simulink model "x3_myfoc_transform"  (R2025b)
settings: Solver=ode23t  StartTime=0.0  StopTime=2  FixedStep=my_Ts  RelTol=1e-3
values from neighbouring files (symbols this model uses):
  Jx = 0.0000005    (= 5e-07)    [foc_para.m]
  Tpwm = 4000-1    (= 3999)    [foc_para.m]
  Ts = 1/SwitchFrequency    (= 5e-05)    [foc_para.m]
  vbus = 12    [foc_para.m]
undefined symbols (not defined in the file or in its folder): DiscIntNeverNeededParam, my_Ts
libraries: ee_lib x11, fl_lib x9, nesl_utility x9, simulink x1
settings Model: Creator=disnox  LastModifiedBy=yolo
settings DataIOCC: ReturnWorkspaceOutputs=off
settings DebuggingCC: SaveWithParameterizedLinksMsg=none  ParameterPrecisionLossMsg=none
settings HardwareCC: ProdBitPerPointer=32.0  ProdBitPerSizeT=32.0  ProdBitPerPtrDiffT=32.0  ProdLargestAtomicInteger=Long  ProdLargestAtomicFloat=Double  ProdWordSize=32.0  ProdHWDeviceType=ARM Compatible->ARM Cortex-M
settings RTWCC: GPUComputeCapability=3.5

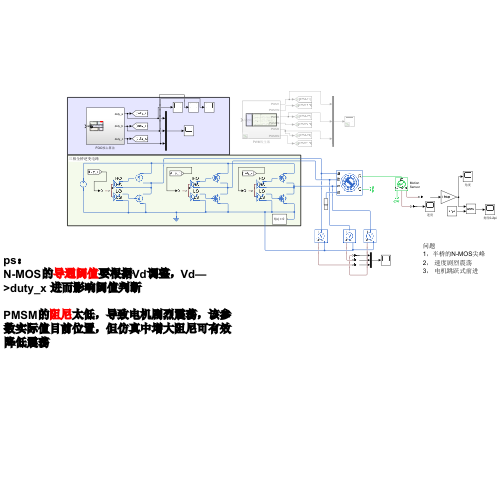
[thumbnail: Simulink's stored preview of the top-level diagram]
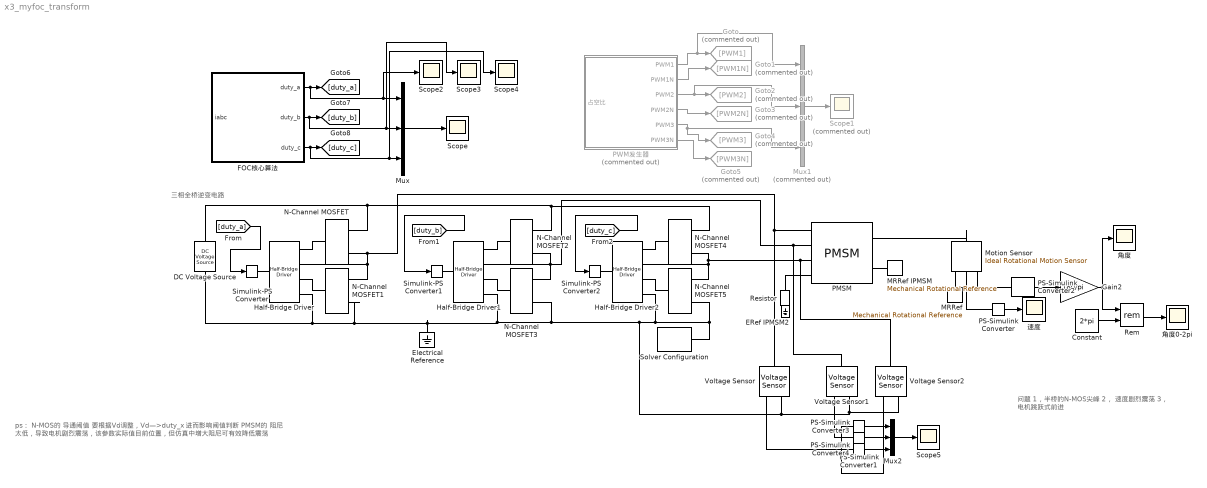
== system x3_myfoc_transform ==
  note: 问题
      | 1，半桥的N-MOS尖峰
      | 2， 速度剧烈震荡
      | 3， 电机跳跃式前进
  note: ps：
      | N-MOS的 导通阈值 要根据Vd调整，Vd—>duty_x 进而影响阈值判断
      |
      | PMSM的 阻尼 太低，导致电机剧烈震荡，该参数实际值目前位置，但仿真中增大阻尼可有效降低震荡
  note: 三相全桥逆变电路
  Constant : Constant  Value=2*pi
  DC Voltage Source : ee_lib/Additional Components/SPICE Sources/DC Voltage Source  DC=12 V
  ERef IPMSM2 : fl_lib/Electrical/Electrical Elements/Electrical Reference
  Electrical Reference : fl_lib/Electrical/Electrical Elements/Electrical Reference
  FOC核心算法 : Subsystem
  Gain2 : Gain  Gain=180/pi
  Goto : Goto  Commented=on  GotoTag=PWM1
  Goto1 : Goto  Commented=on  GotoTag=PWM1N
  Goto2 : Goto  Commented=on  GotoTag=PWM2
  Goto3 : Goto  Commented=on  GotoTag=PWM2N
  Goto4 : Goto  Commented=on  GotoTag=PWM3
  Goto5 : Goto  Commented=on  GotoTag=PWM3N
  Half-Bridge Driver : ee_lib/Semiconductors & Converters/Half-Bridge Driver  port_option=ee.enum.controlport.ps  uHigh=2.0 V  uLow=0.8 V  uHighValue=0.6  uLowValue=0.4  vHigh=12 V  vLow=0 V  tpLH=50 ns  tdLH=5 us  tpHL=50 ns  tdHL=5 us  parameterization=ee.enum.semiconductors.gateDriverParam.outputImpedance  rHigh=50 Ohm  rLow=50 Ohm  tRise=20 ns  tFall=20 ns  cLoad=10 nF  ZonTime_specify=off  ZonTime_priority=None  ZonTime=0 s  ZoffTime_specify=off  ZoffTime_priority=None  ZoffTime=0 s  power_dissipated_high_side_specify=off  power_dissipated_high_side_priority=None  power_dissipated_high_side=0 W  power_dissipated_high_side_nominal_specify=off  power_dissipated_high_side_nominal_value=1  power_dissipated_high_side_nominal_unit=W  power_dissipated_low_side_specify=off  power_dissipated_low_side_priority=None  power_dissipated_low_side=0 W  power_dissipated_low_side_nominal_specify=off  power_dissipated_low_side_nominal_value=1  power_dissipated_low_side_nominal_unit=W
      settings: InternalSimscapePortConfiguration="{\"Bottom\":[],\"Left\":[{\"id\":\"u\",\"label\":\"u\",\"type\":\"input\"}],\"Right\":[{\"id\":\"HO\",\"label\":\"HO\",\"type\":\"foundation.electrical.electrical\"},{\"id\":\"HS\",\"label\":\"HS\",\"type\":\"foundation.electrical.electrical\"},{\"id\":\"LO\",\"label\":\"LO\",\"type\":\"foundation.electrical.electrical\"},{\"id\":\"LS\",\"label\":\"LS\",\"type\":\"foundation.electrical.electrical\"}],\"Top\":[]}"
  Half-Bridge Driver1 : ee_lib/Semiconductors & Converters/Half-Bridge Driver  port_option=ee.enum.controlport.ps  uHigh=2.0 V  uLow=0.8 V  uHighValue=0.6  uLowValue=0.4  vHigh=12 V  vLow=0 V  tpLH=50 ns  tdLH=5 us  tpHL=50 ns  tdHL=5 us  parameterization=ee.enum.semiconductors.gateDriverParam.outputImpedance  rHigh=50 Ohm  rLow=50 Ohm  tRise=20 ns  tFall=20 ns  cLoad=10 nF  ZonTime_specify=off  ZonTime_priority=None  ZonTime=0 s  ZoffTime_specify=off  ZoffTime_priority=None  ZoffTime=0 s  power_dissipated_high_side_specify=off  power_dissipated_high_side_priority=None  power_dissipated_high_side=0 W  power_dissipated_high_side_nominal_specify=off  power_dissipated_high_side_nominal_value=1  power_dissipated_high_side_nominal_unit=W  power_dissipated_low_side_specify=off  power_dissipated_low_side_priority=None  power_dissipated_low_side=0 W  power_dissipated_low_side_nominal_specify=off  power_dissipated_low_side_nominal_value=1  power_dissipated_low_side_nominal_unit=W
      settings: InternalSimscapePortConfiguration="{\"Bottom\":[],\"Left\":[{\"id\":\"u\",\"label\":\"u\",\"type\":\"input\"}],\"Right\":[{\"id\":\"HO\",\"label\":\"HO\",\"type\":\"foundation.electrical.electrical\"},{\"id\":\"HS\",\"label\":\"HS\",\"type\":\"foundation.electrical.electrical\"},{\"id\":\"LO\",\"label\":\"LO\",\"type\":\"foundation.electrical.electrical\"},{\"id\":\"LS\",\"label\":\"LS\",\"type\":\"foundation.electrical.electrical\"}],\"Top\":[]}"
  Half-Bridge Driver2 : ee_lib/Semiconductors & Converters/Half-Bridge Driver  port_option=ee.enum.controlport.ps  uHigh=2.0 V  uLow=0.8 V  uHighValue=0.6  uLowValue=0.4  vHigh=12 V  vLow=0 V  tpLH=50 ns  tdLH=5 us  tpHL=50 ns  tdHL=5 us  parameterization=ee.enum.semiconductors.gateDriverParam.outputImpedance  rHigh=50 Ohm  rLow=50 Ohm  tRise=20 ns  tFall=20 ns  cLoad=10 nF  ZonTime_specify=off  ZonTime_priority=None  ZonTime=0 s  ZoffTime_specify=off  ZoffTime_priority=None  ZoffTime=0 s  power_dissipated_high_side_specify=off  power_dissipated_high_side_priority=None  power_dissipated_high_side=0 W  power_dissipated_high_side_nominal_specify=off  power_dissipated_high_side_nominal_value=1  power_dissipated_high_side_nominal_unit=W  power_dissipated_low_side_specify=off  power_dissipated_low_side_priority=None  power_dissipated_low_side=0 W  power_dissipated_low_side_nominal_specify=off  power_dissipated_low_side_nominal_value=1  power_dissipated_low_side_nominal_unit=W
      settings: InternalSimscapePortConfiguration="{\"Bottom\":[],\"Left\":[{\"id\":\"u\",\"label\":\"u\",\"type\":\"input\"}],\"Right\":[{\"id\":\"HO\",\"label\":\"HO\",\"type\":\"foundation.electrical.electrical\"},{\"id\":\"HS\",\"label\":\"HS\",\"type\":\"foundation.electrical.electrical\"},{\"id\":\"LO\",\"label\":\"LO\",\"type\":\"foundation.electrical.electrical\"},{\"id\":\"LS\",\"label\":\"LS\",\"type\":\"foundation.electrical.electrical\"}],\"Top\":[]}"
  MRRef : fl_lib/Mechanical/Rotational Elements/Mechanical Rotational Reference
  MRRef IPMSM : fl_lib/Mechanical/Rotational Elements/Mechanical Rotational Reference
  Motion Sensor : fl_lib/Mechanical/Mechanical Sensors/Ideal Rotational Motion Sensor  reference=foundation.enum.MeasurementReference.difference  acceleration_port=false  velocity_port=true  position_port=true  wrap_angle=false  offset=0 deg
  Mux : Mux  Inputs=3
  Mux1 : Mux  Commented=on  Inputs=3
  Mux2 : Mux  Inputs=3
  N-Channel MOSFET{,1..5} (6 alike) : ee_lib/Semiconductors & Converters/N-Channel MOSFET  paramTerminal=ee.enum.mosfet.numberOfTerminals.three  parameterization=ee.enum.mosfet.parameterization.datasheet  Beta=5.0 A/V^2  Rds=0.025 Ohm  Id=6.0 A  Vgs=10 V  Vth=1.7 V  Vth0=1.7 V  lam=0 1/V  gamma_vth=0.5 V^(1/2)  phib=0.5 V  Vth1=1.9071 V  Vbs1=-1 V  Vth2=2.066 V  Vbs2=-2 V  Tmeas=25 degC  Vgs_vec=[-1, -.5, 2, 3, 4, 5] V  Vds_vec=[0, 2, 4, 8, 12, 16, 20] V  Vbs_vec=[0, -4, -6, -12] V  T_vec=[25, 125] degC  Vth_vec=[.4, 1.2, 1.4, 1.45] V  Vth_mat=[.4, .35; 1.2, 1.15; 1.4, 1.35; 1.45, 1.4] V  Ids_mat=[0, 0, 0, 0, 0, 0, 0; 0, 0, 0, 0, 0, 0, 0; 0, .003, .0038, .0043, .0046, .0048, .0049; 0, .0055, .008, .009, .0095, .01, .0101; 0, .0115, .016, .018, .019, .0195, .02; 0, .0152, .0225, .0265, .028, .0295, .03] A  Ids_mat0=[0, 0, 0, 0, 0, 0, 0; 0, 0, 0, 0, 0, 0, 0; 0, .003, .0038, .0043, .0046, .0048, .0049; 0, .0055, .008, .009, .0095, .01, .0101; 0, .0115, .016, .018, .019, .0195, .02; 0, .0152, .0225, .0265, .028, .0295, .03] A  Ids_mat_3D=zeros(6, 7, 2) A  Ids_mat_3D0=zeros(6, 7, 2) A  IV_table_symmetry=ee.enum.mosfet.symmetricNIV.no  RS=0.0001 Ohm  RD=0.01 Ohm  RB=0.001 Ohm  LeadRs=0 Ohm  LeadRd=0 Ohm  LeadRg=0 Ohm  LeadRb=0 Ohm  LS=0 nH  LD=0 nH  LG=0 nH  LB=0 nH  C_param=ee.enum.mosfet.capacitanceParam.fixedciss  C_GS=270 pF  C_GD=80 pF  C_GB=0 pF  C_DS=0 pF  C_iss=350 pF  C_rss=80 pF  C_oss=0 pF  C_iss_vec=[720, 700, 590, 470, 390, 310] pF  C_rss_vec=[450, 400, 300, 190, 95, 55] pF  C_oss_vec=[900, 810, 690, 420, 270, 170] pF  C_GS_vec=[270, 300, 290, 280, 295, 255] pF  C_GD_vec=[450, 400, 300, 190, 95, 55] pF  C_GB_vec=[270, 300, 290, 280, 295, 255] pF  C_Vgs_vec=0 V  C_DS_vec=[450, 410, 390, 230, 175, 115] pF  C_Vds_vec=[.1, .3, 1, 3, 10, 30] V  V_GS_for_cap_data=0 V  charge_linearity_param=ee.enum.mosfet.cgdLinearity.constant  C_OX=200 pF  V_C_OX=-0.5 V  charge_linearity_param_vgb=ee.enum.mosfet.cgbLinearity.instantly  charge_linearity_param_with_vgb=ee.enum.mosfet.cgbLinearityWithSeparateCgb.instantly  Di_param=ee.enum.mosfet.diodeParam.no  IsDiode=1e-12 A  Vbi=0.6 V  n=1  Cj0Diode=0 pF  TT=50e-9 s  Tmeas_dio=25 degC  TableTypeNoT=ee.enum.mosfet.tableType.IfMat  TableType=ee.enum.diode.tableType.IfMat  IfVec=[.07, .12, .19, 1.75, 4.24, 7.32, 11.2] A  IfMat=[.07, .12, .19, 1.75, 4.24, 7.32, 11.2; .16, .3, .72, 2.14, 4.02, 6.35, 9.12] A  VfVecV=[.9, 1.15, 1.25, 1.5, 1.75, 2.17, 2.6, 2.85] V  VfMatV=[.9, 1.15, 1.25, 1.5, 1.75, 2.17, 2.6, 2.85; .58, .68, .75, 1.1, 1.38, 1.77, 2.27, 2.7] V  TjVec=[25, 125] degC  VfVec=[.5, .7, .9, 1.3, 1.7, 2.1, 2.5] V  IfVecV=[.1, .2, .5, 1, 2, 4, 7, 10] A  diode_Goff=1e-12 1/Ohm  prmDatasheet=ee.enum.temperatureParameterization.none  prmEquCoeff=ee.enum.temperatureParameterization.none  dVth_dT=-6 mV/K  dVth0_dT=-6 mV/K  Rds_T2=0.037 Ohm  BEXDatasheet=-1.5  BEXEquCoeff=-1.5  etaisDatasheet=3  etaisEquCoeff=3  Tmeas2=125 degC  etaisTabulated=3  TdeviceDatasheet=25 degC  TdeviceEquCoeff=25 degC  TdeviceTabulated=25 degC  i_g_specify=off  i_g_priority=None  i_g=0 A  i_g_nominal_specify=off  i_g_nominal_value=1  i_g_nominal_unit=A  i_d_specify=off  i_d_priority=None  i_d=0 A  i_d_nominal_specify=off  i_d_nominal_value=1  i_d_nominal_unit=A  i_b_specify=off  i_b_priority=None  i_b=0 A  i_b_nominal_specify=off  i_b_nominal_value=1  i_b_nominal_unit=A  voltage_gs_specify=off  voltage_gs_priority=None  voltage_gs=0 V  voltage_gs_nominal_specify=off  voltage_gs_nominal_value=1  voltage_gs_nominal_unit=V  voltage_ds_specify=off  voltage_ds_priority=None  voltage_ds=0 V  voltage_ds_nominal_specify=off  voltage_ds_nominal_value=1  voltage_ds_nominal_unit=V  voltage_bs_specify=off  voltage_bs_priority=None  voltage_bs=0 V  voltage_bs_nominal_specify=off  voltage_bs_nominal_value=1  voltage_bs_nominal_unit=V  v_Cgs_specify=off  v_Cgs_priority=High  v_Cgs=0 V  v_Cgs_nominal_specify=off  v_Cgs_nominal_value=1  v_Cgs_nominal_unit=V  v_Cds_specify=off  v_Cds_priority=High  v_Cds=0 V  v_Cds_nominal_specify=off  v_Cds_nominal_value=1  v_Cds_nominal_unit=V  v_Cbs_specify=off  v_Cbs_priority=High  v_Cbs=0 V  v_Cbs_nominal_specify=off  v_Cbs_nominal_value=1  v_Cbs_nominal_unit=V  thermal_network_parameterization=ee.enum.thermalNetworkTopology.junctionCase  Rth=[0, 10] K/W  Rth_Cauer=[1, 3, 10] K/W  Rth_Foster=[.08, .14, .22, .16] K/W  thermal_mass_parameterization=ee.enum.thermalNetwork.timeconstant  thermal_mass=[0, 1] J/K  thermal_mass_Cauer=[.1, .3, 1] J/K  thermal_mass_Foster=[.001, .005, .05, .5] J/K  thermal_time_constant=[0, 10] s  thermal_time_constant_Cauer=[1, 3, 10] s  thermal_time_constant_Foster=[7e-05, .0007, .01, .08] s  thermal_mass_initial_temperatures=[25, 25] degC  thermal_mass_initial_temperatures_Cauer=[25, 25, 25] degC  Tvec_initial_Foster=[25, 25, 25, 25] degC  betaref=18 A/V^2  Vfbref=-1.1 V  gamma=3.5 V^(1/2)  phib2ref=1 V  thesatref=0.4 1/V  alpha=0  Vp=5e-2 V  thesrref=0 1/V  m=8  Tref=25 degC  Rsref=2e-3 Ohm  Rdref=0.17 Ohm  Rgref=8.4 Ohm  Rbref=2e-3 Ohm  Cox=1500 pF  Cgso=100 pF  Cgdo=14 pF  Isref=5.2e-13 A  Cj0=480 pF  Tprm=1  etabet=1.3  Stvfb=5e-4 V/K  Stphib=-8.5e-4 V/K  etasat=1.04  etasr=0.65  etar=0.95  etais=3  Tsim=25 degC  Ig_specify=off  Ig_priority=None  Ig=0 A  Ig_nominal_specify=off  Ig_nominal_value=1  Ig_nominal_unit=nA  Ids_specify=off  Ids_priority=None  Ids=0 A  Ids_nominal_specify=off  Ids_nominal_value=1  Ids_nominal_unit=A  Ib_specify=off  Ib_priority=None  Ib=0 A  Ib_nominal_specify=off  Ib_nominal_value=1  Ib_nominal_unit=uA  V_gs_specify=off  V_gs_priority=None  V_gs=0 V  V_gs_nominal_specify=off  V_gs_nominal_value=1  V_gs_nominal_unit=V  V_ds_specify=off  V_ds_priority=None  V_ds=0 V  V_ds_nominal_specify=off  V_ds_nominal_value=1  V_ds_nominal_unit=V  V_bs_specify=off  V_bs_priority=None  V_bs=0 V  V_bs_nominal_specify=off  V_bs_nominal_value=1  V_bs_nominal_unit=V  QGoverCox_specify=off  QGoverCox_priority=None  QGoverCox=0 V  QGoverCox_nominal_specify=off  QGoverCox_nominal_value=1  QGoverCox_nominal_unit=V  QDoverCox_specify=off  QDoverCox_priority=None  QDoverCox=0 V  QDoverCox_nominal_specify=off  QDoverCox_nominal_value=1  QDoverCox_nominal_unit=V  QBoverCox_specify=off  QBoverCox_priority=None  QBoverCox=0 V  QBoverCox_nominal_specify=off  QBoverCox_nominal_value=1  QBoverCox_nominal_unit=V  T0=[25, 25] degC  T0_Cauer=[25, 25, 25] degC
  PMSM : ee_lib/Electromechanical/Permanent Magnet/PMSM  port_option=ee.enum.threePhasePort.expanded  winding_type=ee.enum.electromech.statorconfiguration.wye  machine_param=ee.enum.pmsm.parameterization.constant  nPolePairs=Np  pmflux_param=ee.enum.pmflux.fluxlinkage  pm_flux_linkage=Flux Wb  torque_constant=0.18 N*m/A  back_emf_constant=0.18 V*s/rad  stator_param=ee.enum.statorparam.LdLqL0  Ld=Ld H  Lq=Lq H  idVec=[-200, 0, 200] A  iqVec=[-200, 0, 200] A  LdMatrix=0.0002 * ones(3, 3) H  LqMatrix=0.0002 * ones(3, 3) H  PmMatrix=0.1 * ones(3, 3) Wb  ktMatrix=0.18 * ones(3, 3) N*m/A  keMatrix=0.18 * ones(3, 3) V*s/rad  L0=0.00016 H  Ls=0.0002 H  Lm=-0.00002 H  Ms=0.00002 H  Rs=Rs Ohm  zero_sequence=ee.enum.park.zerosequence.include  axes_param=ee.enum.rotorangle.daxis  loss_param=ee.enum.ironloss.none  losses_oc=[0, 0, 0] W  losses_sc=[0, 0, 0] W  f_losses=60 Hz  Isc_losses=95 A  J=Jx kg*m^2  lam=0.001 N*m*s/rad  i_d_specify=off  i_d_priority=None  i_d=0 A  i_d_nominal_specify=off  i_d_nominal_value=1  i_d_nominal_unit=A  i_q_specify=off  i_q_priority=None  i_q=0 A  i_q_nominal_specify=off  i_q_nominal_value=1  i_q_nominal_unit=A  torque_specify=off  torque_priority=None  torque=0 N*m  torque_nominal_specify=off  torque_nominal_value=1  torque_nominal_unit=N*m  angular_velocity_specify=off  angular_velocity_priority=High  angular_velocity=0 rpm  angular_velocity_nominal_specify=off  angular_velocity_nominal_value=1  angular_velocity_nominal_unit=rpm  angular_position_specify=off  angular_position_priority=High  angular_position=0 deg  angular_position_nominal_specify=off  angular_position_nominal_value=1  angular_position_nominal_unit=deg  alpha=3.93e-3 1/K  alpha_flux=-0.001 1/K  Tmeas=298.15 K  stator_thermal_mass=100 J/K  rotor_thermal_mass=200 J/K  Rm_percent_rotor=90  Rd_percent_rotor=30  temperatureA_specify=off  temperatureA_priority=High  temperatureA=25 degC  temperatureA_nominal_specify=off  temperatureA_nominal_value=1  temperatureA_nominal_unit=degC  temperatureB_specify=off  temperatureB_priority=High  temperatureB=25 degC  temperatureB_nominal_specify=off  temperatureB_nominal_value=1  temperatureB_nominal_unit=degC  temperatureC_specify=off  temperatureC_priority=High  temperatureC=25 degC  temperatureC_nominal_specify=off  temperatureC_nominal_value=1  temperatureC_nominal_unit=degC  temperatureR_specify=off  temperatureR_priority=High  temperatureR=25 degC  temperatureR_nominal_specify=off  temperatureR_nominal_value=1  temperatureR_nominal_unit=degC
      settings: InternalSimscapePortConfiguration="{\"Bottom\":[],\"Left\":[{\"id\":\"a\",\"label\":\"a\",\"type\":\"foundation.electrical.electrical\"},{\"id\":\"b\",\"label\":\"b\",\"type\":\"foundation.electrical.electrical\"},{\"id\":\"c\",\"label\":\"c\",\"type\":\"foundation.electrical.electrical\"},{\"id\":\"n\",\"label\":\"n\",\"type\":\"foundation.electrical.electrical\"}],\"Right\":[{\"id\":\"R\",\"label\":\"R\",\"type\":\"foundation.mechanical.rotational.rotational\"},{\"id\":\"C\",\"label\":\"C\",\"type\":\"foundation.mechanical.rotational.rotational\"}],\"Top\":[]}"
  PS-Simulink Converter : nesl_utility/PS-Simulink Converter  PhysicalDomain=network_engine_domain  SubClassName=ps_output  LeftPortType=input  RightPortType=output  PseudoPeriodic=off  Frequencies=[]  VectorFormat=inherit  Unit=rad/s  AffineConversion=off
  PS-Simulink Converter1 : nesl_utility/PS-Simulink Converter  PhysicalDomain=network_engine_domain  SubClassName=ps_output  LeftPortType=input  RightPortType=output  PseudoPeriodic=off  Frequencies=[]  VectorFormat=inherit  Unit=inherit  AffineConversion=off
  PS-Simulink Converter2 : nesl_utility/PS-Simulink Converter  PhysicalDomain=network_engine_domain  SubClassName=ps_output  LeftPortType=input  RightPortType=output  PseudoPeriodic=off  Frequencies=[]  VectorFormat=1-D array  Unit=rad  AffineConversion=off
  PS-Simulink Converter3 : nesl_utility/PS-Simulink Converter  PhysicalDomain=network_engine_domain  SubClassName=ps_output  LeftPortType=input  RightPortType=output  PseudoPeriodic=off  Frequencies=[]  VectorFormat=inherit  Unit=inherit  AffineConversion=off
  PS-Simulink Converter4 : nesl_utility/PS-Simulink Converter  PhysicalDomain=network_engine_domain  SubClassName=ps_output  LeftPortType=input  RightPortType=output  PseudoPeriodic=off  Frequencies=[]  VectorFormat=inherit  Unit=inherit  AffineConversion=off
  PWM发生器 : Subsystem  Commented=on
  Rem : Math  Operator=rem
  Resistor : fl_lib/Electrical/Electrical Elements/Resistor  R=1e9 Ohm  i_specify=off  i_priority=None  i=0 A  i_nominal_specify=off  i_nominal_value=1  i_nominal_unit=A  v_specify=off  v_priority=None  v=0 V  v_nominal_specify=off  v_nominal_value=1  v_nominal_unit=V
  Scope{,2..5} (5 alike) : Scope
      Scope settings: ActiveDisplayYMinimum=0.31957804087824193  ActiveDisplayYMaximum=0.68042195912175807  DataLoggingVariableName=ScopeData15
      Scope2 settings: ActiveDisplayYMinimum=-0.37624405782146064  ActiveDisplayYMaximum=1.3678304816261502  DataLoggingVariableName=ScopeData17
      Scope3 settings: ActiveDisplayYMinimum=-0.24057027373037865  ActiveDisplayYMaximum=1.4204530971721079  DataLoggingVariableName=ScopeData18
      Scope4 settings: ActiveDisplayYMinimum=-0.24057027373037865  ActiveDisplayYMaximum=1.4204530971721079  DataLoggingVariableName=ScopeData19
      Scope5 settings: ActiveDisplayYMinimum=-9.0067395854845973  ActiveDisplayYMaximum=21.007224453015507  DataLoggingVariableName=ScopeData21
  Scope1 : Scope  Commented=on
      settings: DataLoggingVariableName=ScopeData14
  Simulink-PS Converter : nesl_utility/Simulink-PS Converter  PhysicalDomain=network_engine_domain  SubClassName=ps_input  LeftPortType=input  RightPortType=output  PseudoPeriodic=off  Frequencies=[]  NoiseDistribution=none  NoiseParameters=[]  Unit=1  AffineConversion=off  FilteringAndDerivatives=provide  SimscapeFilterOrder=1  InputFilterTimeConstant=0.001  UdotUserProvided=0
  Simulink-PS Converter1 : nesl_utility/Simulink-PS Converter  PhysicalDomain=network_engine_domain  SubClassName=ps_input  LeftPortType=input  RightPortType=output  PseudoPeriodic=off  Frequencies=[]  NoiseDistribution=none  NoiseParameters=[]  Unit=1  AffineConversion=off  FilteringAndDerivatives=provide  SimscapeFilterOrder=1  InputFilterTimeConstant=0.001  UdotUserProvided=0
  Simulink-PS Converter2 : nesl_utility/Simulink-PS Converter  PhysicalDomain=network_engine_domain  SubClassName=ps_input  LeftPortType=input  RightPortType=output  PseudoPeriodic=off  Frequencies=[]  NoiseDistribution=none  NoiseParameters=[]  Unit=1  AffineConversion=off  FilteringAndDerivatives=provide  SimscapeFilterOrder=1  InputFilterTimeConstant=0.001  UdotUserProvided=0
  Solver Configuration : nesl_utility/Solver Configuration  PhysicalDomain=network_engine_domain  SubClassName=solver  LeftPortType=input  RightPortType=generic  Tones=[]  Harmonics=[]  SimulateNoise=off  Profile=off  UseLocalSampling=off  EnableSwitchedLinearOptims=on  FrequencyDomain=off  UseCCode=off  RelTol=0.001  AbsTol=0.001  MinStep=1e-09  ToWorkspace=off  RevertToSquareIcSolve=off  NumHomotopyIterations=100  PhasorMode=off  PhasorModeNumHarmonics=1  ConsistencySolver=NEWTON_XTOL_AFTER_FTOL  IndexReductionMethod=DerivativeReplacement  DoDC=off  ResidualTolerance=1e-09  ConsistencyTolSource=GLOBAL  ConsistencyAbsTol=0.001  ConsistencyRelTol=0.001  ConsistencyTolFactor=0.001  UseLocalSolver=off  LocalSolverChoice=NE_BACKWARD_EULER_ADVANCER  ResolveIndetEquations=on  FunctionEvalNumThread=1  LocalSolverSampleTime=0.001  DoFixedCost=off  MaxNonlinIter=3  MaxModeIter=2  ComputeImpulses=off  ImpulseIterations=2  LinearAlgebra=auto  LinearAlgebraNumThread=0  EquationFormulation=NE_TIME_EF  DelaysMemoryBudget=1024  AutomaticFiltering=on  FilteringTimeConstant=0.001  PartitionStorageMethod=AS_NEEDED  PartitionMemoryBudget=1024  PartitionMethod=ROBUST  MultibodyUseLocalSolver=off  MultibodyLocalSolverChoice=ODE1  MultibodyLocalSolverSampleTime=0.001
  Voltage Sensor : fl_lib/Electrical/Electrical Sensors/Voltage Sensor
  Voltage Sensor1 : fl_lib/Electrical/Electrical Sensors/Voltage Sensor
  Voltage Sensor2 : fl_lib/Electrical/Electrical Sensors/Voltage Sensor
  角度 : Scope
      settings: ActiveDisplayYMinimum=-209.56347973664643  ActiveDisplayYMaximum=1705.709687460886  DataLoggingVariableName=ScopeData13
  角度0-2pi : Scope
      settings: ActiveDisplayYMinimum=-7.8029507256515176  ActiveDisplayYMaximum=7.8481762516138458  DataLoggingVariableName=ScopeData22
  速度 : Scope
      settings: ActiveDisplayYMinimum=-212.28997736456884  ActiveDisplayYMaximum=152.2117262239781  DataLoggingVariableName=ScopeData16
  wires:
  PWM发生器/1(PWM1) -> Mux1/1, Goto/1
  PWM发生器/2(PWM1N) -> Goto1/1
  PWM发生器/3(PWM2) -> Mux1/2, Goto2/1
  PWM发生器/4(PWM2N) -> Goto3/1
  PWM发生器/5(PWM3) -> Goto4/1, Mux1/3
  PWM发生器/6(PWM3N) -> Goto5/1
  Gain2/1 -> Rem/1, 角度/1
  PS-Simulink Converter2/1 -> Gain2/1
  FOC核心算法/1(duty_a) -> Scope2/1, Mux/1, [duty_a]
  FOC核心算法/2(duty_b) -> Scope3/1, Mux/2, [duty_b]
  FOC核心算法/3(duty_c) -> Scope4/1, Mux/3, [duty_c]
  [duty_a] -> Simulink-PS Converter/1
  [duty_b] -> Simulink-PS Converter1/1
  [duty_c] -> Simulink-PS Converter2/1
  Mux/1 -> Scope/1
  Mux1/1 -> Scope1/1
  PS-Simulink Converter/1 -> 速度/1
  Constant/1 -> Rem/2
  Rem/1 -> 角度0-2pi/1
  PS-Simulink Converter4/1 -> Mux2/3
  PS-Simulink Converter1/1 -> Mux2/2
  PS-Simulink Converter3/1 -> Mux2/1
  Mux2/1 -> Scope5/1
  connections:
  Simulink-PS Converter/RConn1 -- Half-Bridge Driver/LConn1
  Half-Bridge Driver/RConn1 -- N-Channel MOSFET/LConn1
  Half-Bridge Driver/RConn2 -- N-Channel MOSFET1/RConn1 -- PMSM/LConn1 -- Voltage Sensor/LConn1 -- N-Channel MOSFET/RConn2
  Half-Bridge Driver/RConn3 -- N-Channel MOSFET1/LConn1
  N-Channel MOSFET/RConn1 -- DC Voltage Source/LConn1 -- N-Channel MOSFET4/RConn1 -- N-Channel MOSFET2/RConn1
  Half-Bridge Driver1/RConn2 -- Voltage Sensor1/LConn1 -- PMSM/LConn2 -- N-Channel MOSFET3/RConn1 -- N-Channel MOSFET2/RConn2
  N-Channel MOSFET1/RConn2 -- Electrical Reference/LConn1 -- Voltage Sensor2/RConn2 -- Voltage Sensor1/RConn2 -- Voltage Sensor/RConn2 -- N-Channel MOSFET5/RConn2 -- Solver Configuration/RConn1 -- Half-Bridge Driver2/RConn4 -- N-Channel MOSFET3/RConn2 -- Half-Bridge Driver1/RConn4 -- DC Voltage Source/RConn1 -- Half-Bridge Driver/RConn4
  Half-Bridge Driver1/RConn1 -- N-Channel MOSFET2/LConn1
  Half-Bridge Driver1/RConn3 -- N-Channel MOSFET3/LConn1
  Half-Bridge Driver1/LConn1 -- Simulink-PS Converter1/RConn1
  Half-Bridge Driver2/RConn2 -- Voltage Sensor2/LConn1 -- PMSM/LConn3 -- N-Channel MOSFET4/RConn2 -- N-Channel MOSFET5/RConn1
  Half-Bridge Driver2/RConn3 -- N-Channel MOSFET5/LConn1
  Half-Bridge Driver2/LConn1 -- Simulink-PS Converter2/RConn1
  Half-Bridge Driver2/RConn1 -- N-Channel MOSFET4/LConn1
  ERef IPMSM2/LConn1 -- Resistor/RConn1
  PMSM/LConn4 -- Resistor/LConn1
  MRRef IPMSM/LConn1 -- PMSM/RConn2
  MRRef/LConn1 -- Motion Sensor/RConn1
  Motion Sensor/RConn3 -- PS-Simulink Converter2/LConn1
  Motion Sensor/LConn1 -- PMSM/RConn1
  PS-Simulink Converter/LConn1 -- Motion Sensor/RConn2
  Voltage Sensor/RConn1 -- PS-Simulink Converter4/LConn1
  Voltage Sensor1/RConn1 -- PS-Simulink Converter1/LConn1
  Voltage Sensor2/RConn1 -- PS-Simulink Converter3/LConn1

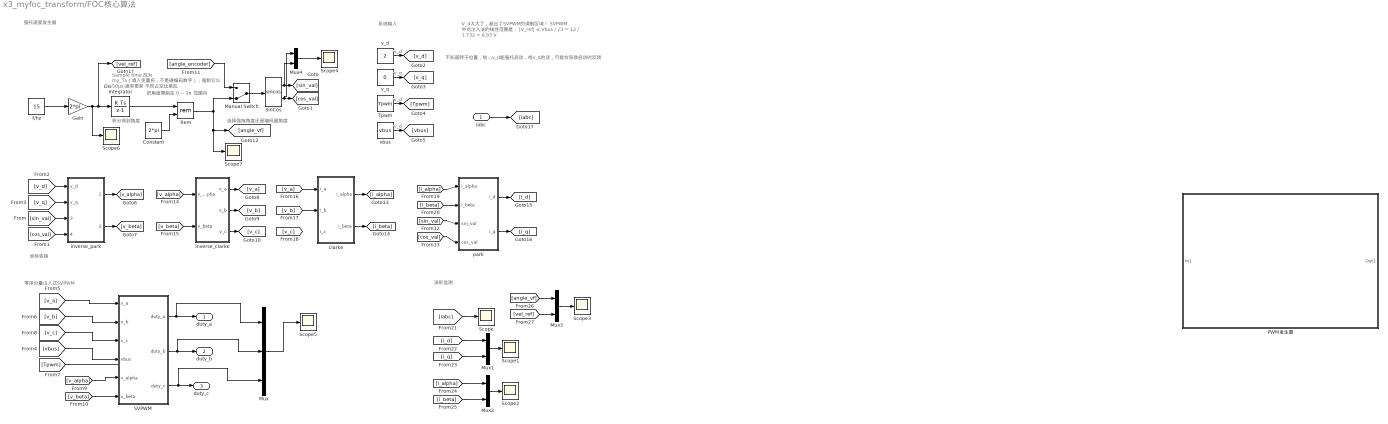
== system x3_myfoc_transform/FOC核心算法 ==
  note: Sample time 改为 my_Ts（填入变量名，不是硬编码数字），强制它以 50μs 速率更新 不然占空比紊乱
  note: V_d太大了，超出了SVPWM的调制区域！
      | SVPWM 中点注入法的线性范围是：
      | |V_ref| ≤ Vbus / √3 = 12 / 1.732 = 6.93 V
  note: 波形监测
  note: 坐标变换
  note: 不知道转子位置，给v_d能强托启动，给v_q的话，可能会导致启动时反转
  note: 积分得到角度
  note: 选择强拖角度还是编码器角度
  note: 零序分量注入式SVPWM
  note: 系统输入
  note: 把角度限制在 0 ~ 2π 范围内
  note: 强托速度发生器
  iabc : Inport
  Constant : Constant  Value=2*pi
  Discrete-Time Integrator : DiscreteIntegrator  SampleTime=my_Ts  ICPrevOutput=DiscIntNeverNeededParam  ICPrevScaledInput=DiscIntNeverNeededParam
  Gain : Gain  Gain=2*pi
  Manual Switch : ManualSwitch  CurrentSetting=0
  Mux : Mux  Inputs=3
  Mux{1..4} (4 alike) : Mux  Inputs=2
  PWM发生器 : Subsystem
  Rem : Math  Operator=rem
  SVPWM : Subsystem
  Scope{,1..7} (8 alike) : Scope
      Scope2 settings: DataLoggingVariableName=ScopeData2
      Scope3 settings: ActiveDisplayYMinimum=-1  ActiveDisplayYMaximum=1  DataLoggingVariableName=ScopeData4
      Scope4 settings: ActiveDisplayYMinimum=-1  ActiveDisplayYMaximum=1  DataLoggingVariableName=ScopeData20
      Scope5 settings: ActiveDisplayYMinimum=-0.041265877365274178  ActiveDisplayYMaximum=1.0412658773652741  DataLoggingVariableName=ScopeData10
      Scope6 settings: ActiveDisplayYMinimum=214.15926535897933  ActiveDisplayYMaximum=414.15926535897933  DataLoggingVariableName=ScopeData11
      Scope7 settings: ActiveDisplayYMinimum=-0.7853981633974445  ActiveDisplayYMaximum=7.0685834705770025  DataLoggingVariableName=ScopeData12
  SinCos : Trigonometry  Operator=sincos
  Tpwm : Constant  Value=Tpwm
  clarke : Subsystem  TreatAsAtomicUnit=on
      settings: RTWSystemCode=Nonreusable function  RTWFcnNameOpts=Use subsystem name
  f/hz : Constant  Value=15
  inverse_clarke : Subsystem
  inverse_park : Subsystem
  park : Subsystem  TreatAsAtomicUnit=on
      settings: RTWSystemCode=Nonreusable function  RTWFcnNameOpts=Use subsystem name
  v_d : Constant  Value=2
  v_q : Constant  Value=0
  vbus : Constant  Value=vbus
  duty_a : Outport
  duty_b : Outport  Port=2
  duty_c : Outport  Port=3
  wires:
  [v_c] -> SVPWM/3(v_c)
  SVPWM/3(duty_c) -> duty_c/1, Mux/3
  [cos_val] -> inverse_park/4(cos_val)
  vbus/1 -> [vbus]  "v_d"
  SinCos/1 -> Mux4/2, [sin_val]
  Gain/1 -> Scope6/1, [vel_ref], Discrete-Time Integrator/1
  f/hz/1 -> Gain/1
  [v_b] -> SVPWM/2(v_b)
  Discrete-Time Integrator/1 -> Rem/1
  SinCos/2 -> Mux4/1, [cos_val]
  [v_q] -> inverse_park/2(v_q)
  [sin_val] -> inverse_park/3(sin_val)
  [cos_val] -> park/4(cos_val)
  Constant/1 -> Rem/2
  [Tpwm] -> ?
  inverse_park/1(v_alpha) -> [v_alpha]
  [v_alpha] -> SVPWM/5(v_alpha)
  [v_d] -> inverse_park/1(v_d)
  Tpwm/1 -> [Tpwm]  "v_d"
  v_q/1 -> [v_q]  "v_q"
  [vbus] -> SVPWM/4(vbus)
  v_d/1 -> [v_d]  "v_d"
  [sin_val] -> park/3(sin_val)
  inverse_park/2(v_beta) -> [v_beta]
  [v_a] -> SVPWM/1(v_a)
  SVPWM/2(duty_b) -> duty_b/1, Mux/2
  SVPWM/1(duty_a) -> duty_a/1, Mux/1
  [v_beta] -> SVPWM/6(v_beta)
  Manual Switch/1 -> SinCos/1
  Rem/1 -> [angle_vf], Scope7/1, Manual Switch/2
  [angle_encoder] -> Manual Switch/1
  park/1(i_d) -> [i_d]
  park/2(i_q) -> [i_q]
  clarke/1(i_alpha) -> [i_alpha]
  clarke/2(i_beta) -> [i_beta]
  inverse_clarke/1(v_a) -> [v_a]
  inverse_clarke/2(v_b) -> [v_b]
  inverse_clarke/3(v_c) -> [v_c]
  [v_alpha] -> inverse_clarke/1(v_alpha)
  [v_beta] -> inverse_clarke/2(v_beta)
  [v_a] -> clarke/1(i_a)
  [v_b] -> clarke/2(i_b)
  [i_alpha] -> park/1(i_alpha)
  [i_beta] -> park/2(i_beta)
  iabc/1 -> [iabc]
  [iabc] -> Scope/1
  [i_d] -> Mux1/1
  [i_q] -> Mux1/2
  Mux1/1 -> Scope1/1
  Mux2/1 -> Scope2/1
  [i_alpha] -> Mux2/1
  [i_beta] -> Mux2/2
  [angle_vf] -> Mux3/1
  [vel_ref] -> Mux3/2
  Mux3/1 -> Scope3/1
  Mux/1 -> Scope5/1
  Mux4/1 -> Scope4/1

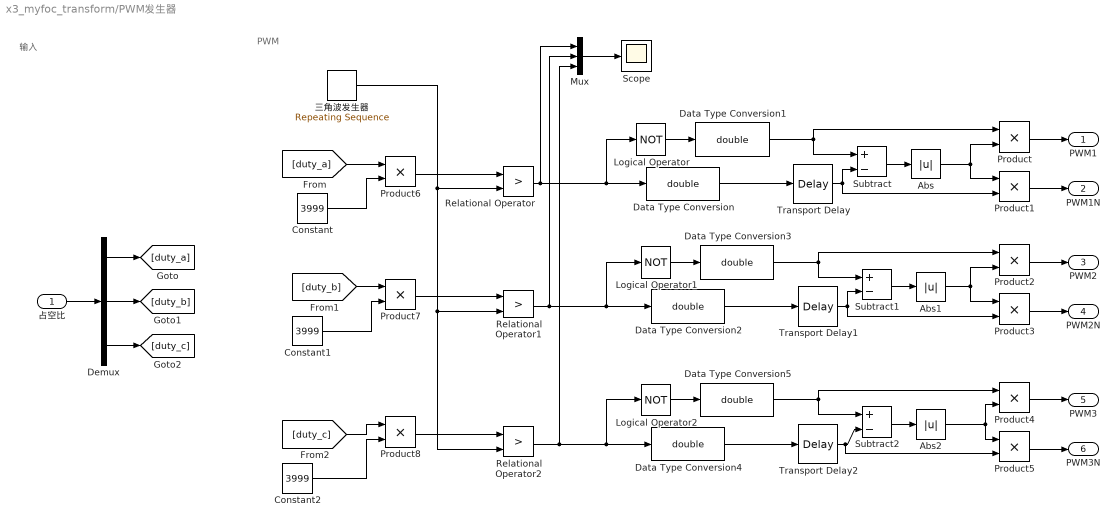
== system x3_myfoc_transform/PWM发生器 ==
  note: PWM
  note: 输入
  占空比 : Inport
  Abs : Abs  SaturateOnIntegerOverflow=off
  Abs1 : Abs  SaturateOnIntegerOverflow=off
  Abs2 : Abs  SaturateOnIntegerOverflow=off
  Constant : Constant  Value=3999
  Constant1 : Constant  Value=3999
  Constant2 : Constant  Value=3999
  Data Type Conversion{,1..5} (6 alike) : DataTypeConversion  OutDataTypeStr=double  SaturateOnIntegerOverflow=off  RndMeth=Floor
  Demux : Demux  Outputs=3
  Logical Operator : Logic  Operator=NOT  AllPortsSameDT=off  OutDataTypeStr=boolean
  Logical Operator1 : Logic  Operator=NOT  AllPortsSameDT=off  OutDataTypeStr=boolean
  Logical Operator2 : Logic  Operator=NOT  AllPortsSameDT=off  OutDataTypeStr=boolean
  Mux : Mux  Inputs=3
  Product{,1..8} (9 alike) : Product
  Relational Operator : RelationalOperator  Operator=>  OutDataTypeStr=boolean  RndMeth=Simplest  InputSameDT=off
  Relational Operator1 : RelationalOperator  Operator=>  OutDataTypeStr=boolean  RndMeth=Simplest  InputSameDT=off
  Relational Operator2 : RelationalOperator  Operator=>  OutDataTypeStr=boolean  RndMeth=Simplest  InputSameDT=off
  Scope : Scope
      settings: ActiveDisplayYMinimum=-0.50570661961685548  ActiveDisplayYMaximum=1.530411663854949  DataLoggingVariableName=ScopeData6
  Subtract : Sum  Inputs=+-
  Subtract1 : Sum  Inputs=+-
  Subtract2 : Sum  Inputs=+-
  Transport Delay : TransportDelay  DelayTime=168/168e6
  Transport Delay1 : TransportDelay  DelayTime=168/168e6
  Transport Delay2 : TransportDelay  DelayTime=168/168e6
  "三角波发生器 " : simulink/Sources/Repeating Sequence  rep_seq_t=[0 Ts/2 Ts]  rep_seq_y=[0 Tpwm 0]
  PWM1 : Outport
  PWM1N : Outport  Port=2
  PWM2 : Outport  Port=3
  PWM2N : Outport  Port=4
  PWM3 : Outport  Port=5
  PWM3N : Outport  Port=6
  wires:
  占空比/1 -> Demux/1
  Demux/1 -> [duty_a]
  Demux/2 -> [duty_b]
  Demux/3 -> [duty_c]
  Logical Operator2/1 -> Data Type Conversion5/1
  Data Type Conversion4/1 -> Transport Delay2/1
  Data Type Conversion/1 -> Transport Delay/1
  Relational Operator1/1 -> Mux/2, Logical Operator1/1, Data Type Conversion2/1
  Logical Operator/1 -> Data Type Conversion1/1
  Transport Delay/1 -> Product1/2, Subtract/2
  Abs2/1 -> Product5/1, Product4/2
  Data Type Conversion1/1 -> Subtract/1, Product/1
  Relational Operator/1 -> Mux/1, Logical Operator/1, Data Type Conversion/1
  Logical Operator1/1 -> Data Type Conversion3/1
  Subtract2/1 -> Abs2/1
  Subtract/1 -> Abs/1
  Product/1 -> PWM1/1
  Data Type Conversion2/1 -> Transport Delay1/1
  Data Type Conversion5/1 -> Subtract2/1, Product4/1
  Transport Delay1/1 -> Product3/2, Subtract1/2
  Abs1/1 -> Product2/2, Product3/1
  Transport Delay2/1 -> Subtract2/2, Product5/2
  Abs/1 -> Product/2, Product1/1
  Subtract1/1 -> Abs1/1
  Data Type Conversion3/1 -> Subtract1/1, Product2/1
  Product1/1 -> PWM1N/1
  Product2/1 -> PWM2/1
  Product3/1 -> PWM2N/1
  Product4/1 -> PWM3/1
  Product5/1 -> PWM3N/1
  "三角波发生器 "/1 -> Relational Operator/2, Relational Operator1/2, Relational Operator2/2
  Relational Operator2/1 -> Data Type Conversion4/1, Logical Operator2/1, Mux/3
  Mux/1 -> Scope/1
  Constant/1 -> Product6/2
  [duty_a] -> Product6/1
  Product6/1 -> Relational Operator/1
  [duty_b] -> Product7/1
  Product7/1 -> Relational Operator1/1
  Constant1/1 -> Product7/2
  Product8/1 -> Relational Operator2/1
  [duty_c] -> Product8/1
  Constant2/1 -> Product8/2

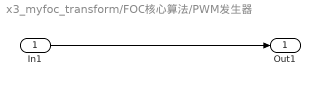
== system x3_myfoc_transform/FOC核心算法/PWM发生器 ==
  In1 : Inport
  Out1 : Outport
  wires:
  In1/1 -> Out1/1

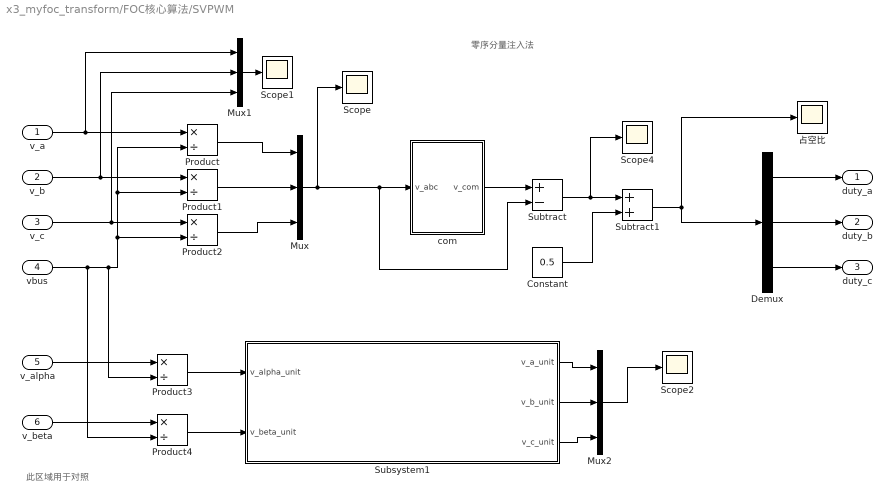
== system x3_myfoc_transform/FOC核心算法/SVPWM ==
  note: 零序分量注入法
  note: 此区域用于对照
  v_a : Inport
  v_b : Inport  Port=2
  v_c : Inport  Port=3
  vbus : Inport  Port=4
  v_alpha : Inport  Port=5
  v_beta : Inport  Port=6
  Constant : Constant  Value=0.5
  Demux : Demux  Outputs=3
  Mux : Mux  Inputs=3
  Mux1 : Mux  Inputs=3
  Mux2 : Mux  Inputs=3
  Product{,1..4} (5 alike) : Product  Inputs=*/
  Scope{,1..2,4} (4 alike) : Scope
      Scope settings: ActiveDisplayYMinimum=-1.0416666666666667  ActiveDisplayYMaximum=1.0416666666666667  DataLoggingVariableName=ScopeData3
      Scope1 settings: ActiveDisplayYMinimum=-12.5  ActiveDisplayYMaximum=12.5  DataLoggingVariableName=ScopeData5
      Scope2 settings: ActiveDisplayYMinimum=-0.10961429555823364  ActiveDisplayYMaximum=0.1562776966292666  DataLoggingVariableName=ScopeData7
      Scope4 settings: ActiveDisplayYMinimum=-0.90210979560879012  ActiveDisplayYMaximum=0.90210979560879012  DataLoggingVariableName=ScopeData9
  Subsystem1 : Subsystem
  Subtract : Sum  Inputs=+-
  Subtract1 : Sum
  com : Subsystem
  占空比 : Scope
      settings: ActiveDisplayYMinimum=-0.40210979560879023  ActiveDisplayYMaximum=1.4021097956087902  DataLoggingVariableName=ScopeData8
  duty_a : Outport
  duty_b : Outport  Port=2
  duty_c : Outport  Port=3
  wires:
  v_a/1 -> Mux1/1, Product/1
  vbus/1 -> Product4/2, Product3/2, Product1/2, Product/2, Product2/2
  v_b/1 -> Mux1/2, Product1/1
  v_c/1 -> Mux1/3, Product2/1
  Product/1 -> Mux/1
  Product1/1 -> Mux/2
  Product2/1 -> Mux/3
  Mux/1 -> Subtract/2, com/1(v_abc), Scope/1
  Mux1/1 -> Scope1/1
  v_alpha/1 -> Product3/1
  v_beta/1 -> Product4/1
  Product3/1 -> Subsystem1/1(v_alpha_unit)
  Product4/1 -> Subsystem1/2(v_beta_unit)
  Subsystem1/1(v_a_unit) -> Mux2/1
  Subsystem1/2(v_b_unit) -> Mux2/2
  Subsystem1/3(v_c_unit) -> Mux2/3
  Mux2/1 -> Scope2/1
  com/1(v_com) -> Subtract/1
  Subtract/1 -> Scope4/1, Subtract1/1
  Constant/1 -> Subtract1/2
  Subtract1/1 -> Demux/1, 占空比/1
  Demux/1 -> duty_a/1
  Demux/2 -> duty_b/1
  Demux/3 -> duty_c/1

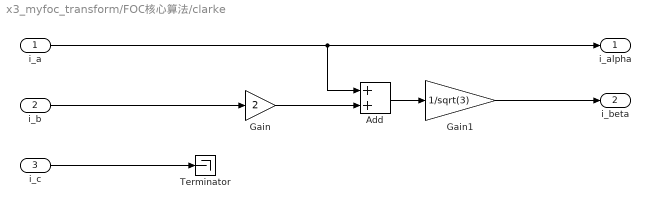
== system x3_myfoc_transform/FOC核心算法/clarke ==
  i_a : Inport
  i_b : Inport  Port=2
  i_c : Inport  Port=3
  Add : Sum
  Gain : Gain  Gain=2
  Gain1 : Gain  Gain=1/sqrt(3)
  Terminator : Terminator
  i_alpha : Outport
  i_beta : Outport  Port=2
  wires:
  i_a/1 -> Add/1, i_alpha/1
  i_b/1 -> Gain/1
  Gain/1 -> Add/2
  Add/1 -> Gain1/1
  Gain1/1 -> i_beta/1
  i_c/1 -> Terminator/1

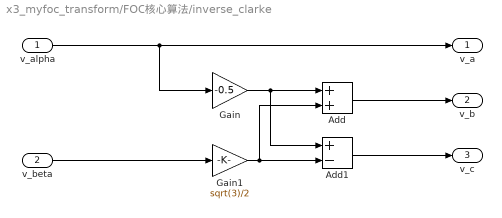
== system x3_myfoc_transform/FOC核心算法/inverse_clarke ==
  v_alpha : Inport
  v_beta : Inport  Port=2
  Add : Sum
  Add1 : Sum  Inputs=+-
  Gain : Gain  Gain=-0.5
  Gain1 : Gain  Gain=sqrt(3)/2
  v_a : Outport
  v_b : Outport  Port=2
  v_c : Outport  Port=3
  wires:
  Gain/1 -> Add1/1, Add/1
  Add1/1 -> v_c/1
  Add/1 -> v_b/1
  Gain1/1 -> Add/2, Add1/2
  v_alpha/1 -> Gain/1, v_a/1
  v_beta/1 -> Gain1/1

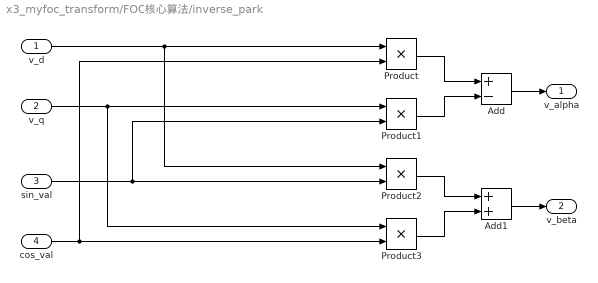
== system x3_myfoc_transform/FOC核心算法/inverse_park ==
  v_d : Inport
  v_q : Inport  Port=2
  sin_val : Inport  Port=3
  cos_val : Inport  Port=4
  Add : Sum  Inputs=+-
  Add1 : Sum  AccumDataTypeStr=double
  Product{,1..3} (4 alike) : Product
  v_alpha : Outport
  v_beta : Outport  Port=2
  wires:
  Add1/1 -> v_beta/1
  v_q/1 -> Product1/1, Product3/1
  Add/1 -> v_alpha/1
  Product/1 -> Add/1
  Product1/1 -> Add/2
  Product2/1 -> Add1/1
  sin_val/1 -> Product2/2, Product1/2
  v_d/1 -> Product2/1, Product/1
  Product3/1 -> Add1/2
  cos_val/1 -> Product3/2, Product/2

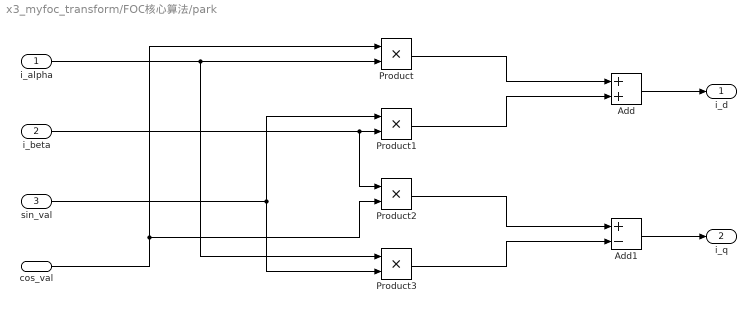
== system x3_myfoc_transform/FOC核心算法/park ==
  i_alpha : Inport
  i_beta : Inport  Port=2
  sin_val : Inport  Port=3
  cos_val : Inport  Port=4
  Add : Sum
  Add1 : Sum  Inputs=+-
  Product{,1..3} (4 alike) : Product
  i_d : Outport
  i_q : Outport  Port=2
  wires:
  i_alpha/1 -> Product/2, Product3/1
  cos_val/1 -> Product2/2, Product/1
  sin_val/1 -> Product3/2, Product1/1
  i_beta/1 -> Product2/1, Product1/2
  Product/1 -> Add/1
  Product1/1 -> Add/2
  Add/1 -> i_d/1
  Product2/1 -> Add1/1
  Product3/1 -> Add1/2
  Add1/1 -> i_q/1

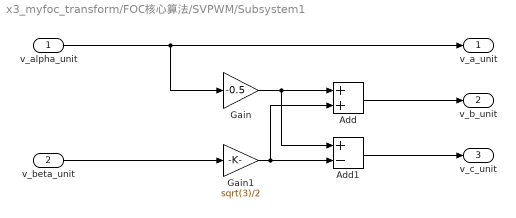
== system x3_myfoc_transform/FOC核心算法/SVPWM/Subsystem1 ==
  v_alpha_unit : Inport
  v_beta_unit : Inport  Port=2
  Add : Sum
  Add1 : Sum  Inputs=+-
  Gain : Gain  Gain=-0.5
  Gain1 : Gain  Gain=sqrt(3)/2
  v_a_unit : Outport
  v_b_unit : Outport  Port=2
  v_c_unit : Outport  Port=3
  wires:
  Gain/1 -> Add1/1, Add/1
  Add1/1 -> v_c_unit/1
  Add/1 -> v_b_unit/1
  Gain1/1 -> Add/2, Add1/2
  v_alpha_unit/1 -> Gain/1, v_a_unit/1
  v_beta_unit/1 -> Gain1/1

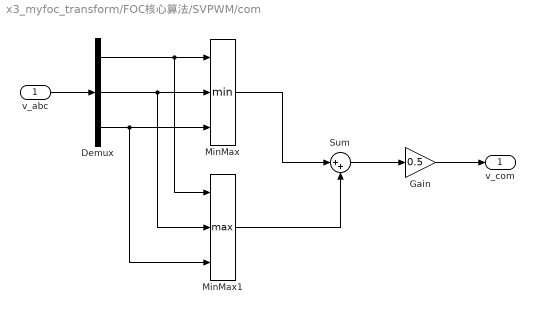
== system x3_myfoc_transform/FOC核心算法/SVPWM/com ==
  v_abc : Inport
  Demux : Demux  Outputs=3
  Gain : Gain  Gain=0.5
  MinMax : MinMax  Inputs=3
  MinMax1 : MinMax  Function=max  Inputs=3
  Sum : Sum  Inputs=|++
  v_com : Outport
  wires:
  v_abc/1 -> Demux/1
  Demux/1 -> MinMax1/1, MinMax/1
  Demux/2 -> MinMax1/2, MinMax/2
  Demux/3 -> MinMax1/3, MinMax/3
  MinMax/1 -> Sum/1
  MinMax1/1 -> Sum/2
  Sum/1 -> Gain/1
  Gain/1 -> v_com/1
